simulink library "carnot"  (R2013b)
settings: Solver=ode45  StartTime=0.0  StopTime=10.0  RelTol=1e-3
undefined symbols (not defined in the file or in its folder): A, acol, Ahabit, Awin, Azimuth_Angle, AziWin, B, C, c1, c4, capc, caph, CarnotCallbacks_Density, CarnotCallbacks_Enthalpy, CarnotCallbacks_Enthalpy2Temperature, CarnotCallbacks_Entropy, CarnotCallbacks_Evaporation_Enthalpy, CarnotCallbacks_GlobalMessageLevel, CarnotCallbacks_Grashof, CarnotCallbacks_Heat_Capacity, CarnotCallbacks_Kinematic_Viscosity, CarnotCallbacks_Prandtl, CarnotCallbacks_Saturation_Property, CarnotCallbacks_Saturation_Temperature, CarnotCallbacks_Saturation_Value_Water, CarnotCallbacks_Specific_Volume, CarnotCallbacks_Thermal_Conductivity, CarnotCallbacks_Vapour_Content, CarnotCallbacks_Vapour_Pressure, con, cond, d, Dd, density, dfin, dia, DiameterLastPiece, DPConstant, dpipe, DPLinear, DPQuadratic, emission_out, fluid, FluidMix, FluidType, FPC, frame, g, GeodeticHeight, Gwin, heat_capacity, hgt, HP, Hroom, ID, inlet, K, l, lin, lpipe ... (+29)
undefined symbols (not defined in the file): c2, c3, c5, c6, cwall, dactive, height, mc, mID, rho, tau, UAneighbour, UAwall, uloss
libraries: carnot x333, simulink x25, simulink_extras x7
(part 9 of 16)

== system carnot/Basic/Material_Properties/Entropy ==
  T : Inport
  p : Inport  Port=2
  Fluid_Type : Inport  Port=3
  Fluid_Mix : Inport  Port=4
  SFunction : S-Function  FunctionName=entroflu  Parameters=DEBUGLEVEL,MAXTOTALMESSAGES,MAXCONSECUTIVEMESSAGES,WRITETOFILE,FILENAME  EnableBusSupport=off
  entropy : Outport
  wires:
  SFunction/1 -> entropy/1
  T/1 -> SFunction/3
  p/1 -> SFunction/4
  Fluid_Type/1 -> SFunction/1
  Fluid_Mix/1 -> SFunction/2

== system carnot/Basic/Material_Properties/Evaporation_Enthalpy ==
  T : Inport
  p : Inport  Port=2
  Fluid_Type : Inport  Port=3
  Fluid_Mix : Inport  Port=4
  SFunction : S-Function  FunctionName=evapoent  Parameters=DEBUGLEVEL,MAXTOTALMESSAGES,MAXCONSECUTIVEMESSAGES,WRITETOFILE,FILENAME  EnableBusSupport=off
  evap_enthalpy : Outport
  wires:
  SFunction/1 -> evap_enthalpy/1
  T/1 -> SFunction/3
  p/1 -> SFunction/4
  Fluid_Type/1 -> SFunction/1
  Fluid_Mix/1 -> SFunction/2

== system carnot/Basic/Material_Properties/Heat_Capacity ==
  T : Inport
  p : Inport  Port=2
  Fluid_Type : Inport  Port=3
  Fluid_Mix : Inport  Port=4
  SFunction : S-Function  FunctionName=capfluid  Parameters=DEBUGLEVEL-1,MAXTOTALWARNINGS,MAXCONSECUTIVEWARNINGS,WRITETOFILE,FILENAME  EnableBusSupport=off
  cp : Outport
  wires:
  SFunction/1 -> cp/1
  T/1 -> SFunction/3
  p/1 -> SFunction/4
  Fluid_Type/1 -> SFunction/1
  Fluid_Mix/1 -> SFunction/2

== system carnot/Basic/Material_Properties/Input_Air ==
  Fluid_mix : Constant  Value=x
  Fluid_type : Constant  Value=2
  Temp : Constant  Value=T
  pres : Constant  Value=p
  Temperature : Outport
  Pressure : Outport  Port=2
  Fluid_type: air : Outport  Port=3
  absolute_humidity : Outport  Port=4
  wires:
  Fluid_mix/1 -> absolute_humidity/1
  Fluid_type/1 -> Fluid_type: air/1
  Temp/1 -> Temperature/1
  pres/1 -> Pressure/1

== system carnot/Basic/Material_Properties/Input_Cotton_Oil ==
  Fluid_mix : Constant  Value=0
  Fluid_type : Constant  Value=3
  Temp : Constant  Value=T
  pres : Constant  Value=p
  Temperature : Outport
  Pressure : Outport  Port=2
  Fluid_cotton_oil : Outport  Port=3
  mix : Outport  Port=4
  wires:
  pres/1 -> Pressure/1
  Temp/1 -> Temperature/1
  Fluid_type/1 -> Fluid_cotton_oil/1
  Fluid_mix/1 -> mix/1

== system carnot/Basic/Material_Properties/Input_Fluid ==
  Fluid_mix_ : Constant  Value=x
  Fluid_type_ : Constant  Value=fluid
  Temp : Constant  Value=T
  pres : Constant  Value=p
  Temperature : Outport
  Pressure : Outport  Port=2
  Fluid_type : Outport  Port=3
  Fluid_mix : Outport  Port=4
  wires:
  pres/1 -> Pressure/1
  Temp/1 -> Temperature/1
  Fluid_type_/1 -> Fluid_type/1
  Fluid_mix_/1 -> Fluid_mix/1

== system carnot/Basic/Material_Properties/Input_Silicon_Oil ==
  Fluid_mix : Constant  Value=0
  Fluid_type : Constant  Value=4
  Temp : Constant  Value=T
  pres : Constant  Value=p
  Temperature : Outport
  Pressure : Outport  Port=2
  Fluid_silicon_oil : Outport  Port=3
  mix : Outport  Port=4
  wires:
  Fluid_mix/1 -> mix/1
  Fluid_type/1 -> Fluid_silicon_oil/1
  Temp/1 -> Temperature/1
  pres/1 -> Pressure/1

== system carnot/Basic/Material_Properties/Input_Tyfocor_LS ==
  Fluid_mix : Constant  Value=0
  Fluid_type : Constant  Value=6
  Temp : Constant  Value=T
  pres : Constant  Value=p
  Temperature : Outport
  Pressure : Outport  Port=2
  Fluid_TyfocorLS : Outport  Port=3
  mix : Outport  Port=4
  wires:
  pres/1 -> Pressure/1
  Temp/1 -> Temperature/1
  Fluid_type/1 -> Fluid_TyfocorLS/1
  Fluid_mix/1 -> mix/1

== system carnot/Basic/Material_Properties/Input_Water ==
  Fluid_mix : Constant  Value=xd
  Fluid_type : Constant
  Temp : Constant  Value=T
  pres : Constant  Value=p
  Temperature : Outport
  Pressure : Outport  Port=2
  Fluid_type: water : Outport  Port=3
  vapour_content : Outport  Port=4
  wires:
  pres/1 -> Pressure/1
  Temp/1 -> Temperature/1
  Fluid_type/1 -> Fluid_type: water/1
  Fluid_mix/1 -> vapour_content/1

== system carnot/Basic/Material_Properties/Input_Water_Glycol ==
  Fluid_mix : Constant  Value=g
  Fluid_type : Constant  Value=5
  Temp : Constant  Value=T
  pres : Constant  Value=p
  Temperature : Outport
  Pressure : Outport  Port=2
  Fluid_type: water/glycol : Outport  Port=3
  "volume content of glycol " : Outport  Port=4
  wires:
  pres/1 -> Pressure/1
  Temp/1 -> Temperature/1
  Fluid_type/1 -> Fluid_type: water/glycol/1
  Fluid_mix/1 -> "volume content of glycol "/1

== system carnot/Basic/Material_Properties/Kinematic_Viscosity ==
  T : Inport
  p : Inport  Port=2
  Fluid_Type : Inport  Port=3
  Fluid_Mix : Inport  Port=4
  SFunction : S-Function  FunctionName=viscous  Parameters=DEBUGLEVEL,MAXTOTALMESSAGES,MAXCONSECUTIVEMESSAGES,WRITETOFILE,FILENAME  EnableBusSupport=off
  visc : Outport
  wires:
  SFunction/1 -> visc/1
  T/1 -> SFunction/3
  p/1 -> SFunction/4
  Fluid_Type/1 -> SFunction/1
  Fluid_Mix/1 -> SFunction/2

== system carnot/Basic/Material_Properties/PhaseCheck ==
  THBin : Inport
  S-Function : S-Function  FunctionName=phasechk  EnableBusSupport=off
  THB2THV : carnot/Toolbox/THB2THV
  wires:
  THBin/1 -> THB2THV/1
  THB2THV/1 -> S-Function/1

== system carnot/Basic/Material_Properties/RelHum2x ==
  note: RG      f · ps
      |  x  = ----  --------------
      |         RD     p - f · ps
      |
      | RG = 287.1 Nm/kgK (Gas Constant Air)
      | RD = 461.5 Nm/kgK (Gas Constant Water Vapour)
      | x absolute Humudity
      | f relative Humidity
      | pD partial pressure of water vapour
  T : Inport
  p : Inport  Port=2
  rel_hum : Inport  Port=3
  Product : Product  Inputs=*/  SaturateOnIntegerOverflow=on  InputSameDT=on  OutDataTypeStr=Inherit: Same as first input
  Product1 : Product  Inputs=*/  SaturateOnIntegerOverflow=on  InputSameDT=on  OutDataTypeStr=Inherit: Same as first input
  Saturation : Saturate  UpperLimit=inf  LowerLimit=0
  Sum : Sum  Inputs=-+  SaturateOnIntegerOverflow=on  InputSameDT=on  OutDataTypeStr=Inherit: Same as first input
  Vapour_Pressure : carnot/Basic/Material_Properties/Vapour_Pressure  VariantControl=CarlibClassic  INPUTARGUMENTS=state variables (classic)  DEBUGLEVEL=WARNINGLEVEL  MAXTOTALMESSAGES=inf  MAXCONSECUTIVEMESSAGES=inf  WRITETOFILE=0  FILENAME='errors.txt'
  mix : Constant  Value=0
  molar mass fraction : Gain  Gain=287.1/461.5  SaturateOnIntegerOverflow=on  OutDataTypeStr=Inherit: Same as input  ParamDataTypeStr=Inherit: Same as input
  p12 : Constant
  percent2absolute : Gain  Gain=0.01  SaturateOnIntegerOverflow=on  OutDataTypeStr=Inherit: Same as input  ParamDataTypeStr=Inherit: Same as input
  water : Constant
  x : Outport
  wires:
  p/1 -> Product/1
  Product/1 -> Sum/2
  Sum/1 -> Product1/2
  Product1/1 -> molar mass fraction/1
  T/1 -> Vapour_Pressure/1
  water/1 -> Vapour_Pressure/3
  p12/1 -> Vapour_Pressure/2
  mix/1 -> Vapour_Pressure/4
  Vapour_Pressure/1 -> Sum/1, Product1/1
  rel_hum/1 -> percent2absolute/1
  percent2absolute/1 -> Product/2
  molar mass fraction/1 -> Saturation/1
  Saturation/1 -> x/1

== system carnot/Basic/Material_Properties/Saturation_Property ==
  T : Inport
  p : Inport  Port=2
  Fluid_Type : Inport  Port=3
  Fluid_Mix : Inport  Port=4
  SFunction : S-Function  FunctionName=satprop  Parameters=PROPERTY, FLUIDPHASE, DEBUGLEVEL, MAXTOTALMESSAGES, MAXCONSECUTIVEMESSAGES, WRITETOFILE, FILENAME  EnableBusSupport=off
  enthalpy : Outport
  wires:
  SFunction/1 -> enthalpy/1
  T/1 -> SFunction/3
  p/1 -> SFunction/4
  Fluid_Type/1 -> SFunction/1
  Fluid_Mix/1 -> SFunction/2

== system carnot/Basic/Material_Properties/Saturation_Temperature ==
  T : Inport
  p : Inport  Port=2
  Fluid_Type : Inport  Port=3
  Fluid_Mix : Inport  Port=4
  SFunction : S-Function  FunctionName=satutemp  Parameters=DEBUGLEVEL,MAXTOTALMESSAGES,MAXCONSECUTIVEMESSAGES,WRITETOFILE,FILENAME  EnableBusSupport=off
  Tsat : Outport
  wires:
  SFunction/1 -> Tsat/1
  T/1 -> SFunction/3
  p/1 -> SFunction/4
  Fluid_Type/1 -> SFunction/1
  Fluid_Mix/1 -> SFunction/2

== system carnot/Basic/Material_Properties/Saturation_Value_Water ==
  T : Inport
  p : Inport  Port=2
  Fluid_Type : Inport  Port=3
  Fluid_Mix : Inport  Port=4
  property_id : Inport  Port=5
  SFunction : S-Function  FunctionName=satprop_vec  Parameters=DEBUGLEVEL,MAXTOTALMESSAGES,MAXCONSECUTIVEMESSAGES,WRITETOFILE,FILENAME  EnableBusSupport=off
  saturation_vapour : Outport
  saturation_liquid : Outport  Port=2
  wires:
  SFunction/1 -> saturation_vapour/1
  SFunction/2 -> saturation_liquid/1
  T/1 -> SFunction/3
  p/1 -> SFunction/4
  Fluid_Type/1 -> SFunction/1
  Fluid_Mix/1 -> SFunction/2
  property_id/1 -> SFunction/5

== system carnot/Basic/Material_Properties/Specific_Volume ==
  T : Inport
  p : Inport  Port=2
  Fluid_Type : Inport  Port=3
  Fluid_Mix : Inport  Port=4
  SFunction : S-Function  FunctionName=specivol  Parameters=DEBUGLEVEL-1,MAXTOTALWARNINGS,MAXCONSECUTIVEWARNINGS,WRITETOFILE,FILENAME  EnableBusSupport=off
  spec_vol : Outport
  wires:
  SFunction/1 -> spec_vol/1
  T/1 -> SFunction/3
  p/1 -> SFunction/4
  Fluid_Type/1 -> SFunction/1
  Fluid_Mix/1 -> SFunction/2

== system carnot/Basic/Material_Properties/THB_Wet_BulbTemperature ==
  THB_air : Inport
  Bus Selector : BusSelector  OutputSignals=Temperature,Pressure,FluidType,FluidMix
  Compare To Constant : simulink/Logic and Bit Operations/Compare To Constant  relop===  const=2  OutDataTypeStr=uint8  ZeroCross=off
  Constant : Constant
  Gain : Gain  Gain=100
  MinMax : MinMax  Inputs=2
  Product : Product  Inputs=*/  RndMeth=Zero
  Product1 : Product  RndMeth=Zero
  Product2 : Product  RndMeth=Zero
  Saturation : Saturate  UpperLimit=100  LowerLimit=0
  Vapour_Pressure1 : carnot/Basic/Material_Properties/Vapour_Pressure  VariantControl=CarlibClassic  INPUTARGUMENTS=state variables (classic)  DEBUGLEVEL=WARNINGLEVEL  MAXTOTALMESSAGES=inf  MAXCONSECUTIVEMESSAGES=inf  WRITETOFILE=0  FILENAME='errors.txt'
  Vapour_Pressure2 : carnot/Basic/Material_Properties/Vapour_Pressure  VariantControl=CarlibClassic  INPUTARGUMENTS=state variables (classic)  DEBUGLEVEL=WARNINGLEVEL  MAXTOTALMESSAGES=inf  MAXCONSECUTIVEMESSAGES=inf  WRITETOFILE=0  FILENAME='errors.txt'
  WBT Fcn of relHum+DBT : Lookup2D  RowIndex=[0,5,10,15,20,25,30,35,40,45,50,55,60,65,70,75,80,85,90,95,100]  ColumnIndex=[-6,-4,-2,0,2,4,6,8,10,12,14,16,18,20,22,24,26,28,30,32,34,36,38,40]  Table=reshape([-10.3,-10.1,-9.9,-9.3,-9.3,-8.9,-8.8,-8.8,-8.3,-8.2,-8.2,-7.7,-7.7,-7.7,-7.1,-7.1,-7.1,-6.6,-6.6,-6.0,-6,-8.3,-8.1,-7.9,-7.9,-7.8,-7.3,-7.3,-6.8,-6.8,-6.7,-6.2,-6.2,-5.7,-5.7,-5.6,-5.1,-5.1,-4.6,-4.6,-4.6,-4,-7.2,-6.9,-6.7,-6.4,-6.1,-5.9,-5.6,-5.3,-5.0,-4.8,-4.8,-4.2,-4.2,-3.7,-3.7,-3.1,-3.1,-2.6,-2.6,-2.6,-2,-5.6,-5.3,-5.0,-5.0,-4.4,-4.4,-3.9,-3.9,-3.3,-3.3,-2.8,-2.8,-2.2,-2.2,-1.7,-1.7,-1.1,-1.1,-0.6,-0.6,0,-4.5,-4.2,-3.9,-3.6,-3.0,-2.8,-2.4,-1.9,-1.9,-1.3,-1.3,-0.8,-0.6,-0.2,0.1,0.4,0.7,1.1,1.4,1.7,2,-3.4,-3.0,-2.7,-2.1,-1.6,-1.1,-1.0,-0.4,0.0,0.1,0.5,0.8,1.2,1.6,1.9,2.3,2.6,3.0,3.3,3.7,4,-1.9,-1.5,-1.1,-0.7,-0.3,0.1,0.5,0.9,1.3,1.8,2.2,2.6,3.0,3.4,3.8,4.1,4.5,4.9,5.3,5.6,6,-0.8,-0.4,0.1,0.6,1.1,1.5,2.0,2.5,2.9,3.4,3.8,4.3,4.7,5.1,5.6,6.0,6.4,6.8,7.2,7.6,8,0.3,0.8,1.4,1.9,2.5,3.0,3.5,4.0,4.5,5.0,5.5,6.0,6.5,6.9,7.4,7.8,8.3,8.7,9.2,9.6,10,1.4,2.1,2.7,3.3,3.9,4.4,5.0,5.6,6.1,6.6,7.2,7.7,8.2,8.7,9.2,9.7,10.2,10.6,11.1,11.6,12,2.6,3.2,3.9,4.6,5.2,5.8,6.5,7.1,7.7,8.2,8.8,9.4,9.9,10.5,11.0,11.5,12.0,12.5,13.0,13.5,14,3.7,4.4,5.1,5.9,6.6,7.3,7.9,8.6,9.2,9.9,10.5,11.1,11.7,12.2,12.8,13.4,13.9,14.5,15.0,15.5,16,4.7,5.5,6.3,7.1,7.9,8.6,9.4,10.1,10.8,11.5,12.1,12.8,13.4,14.0,14.6,15.2,15.8,16.4,16.9,17.5,18,5.7,6.6,7.5,8.4,9.2,10.0,10.8,11.6,12.3,13.1,13.8,14.5,15.1,15.8,16.4,17.1,17.7,18.3,18.9,19.4,20,6.7,7.7,8.7,9.6,10.5,11.4,12.2,13.1,13.9,14.6,15.4,16.1,16.9,17.6,18.2,18.9,19.6,20.2,20.8,21.4,22,7.7,8.8,9.8,10.8,11.8,12.8,13.7,14.6,15.4,16.2,17.0,17.8,18.6,19.3,20.1,20.8,21.4,22.1,22.7,23.4,24,8.6,9.8,11.0,12.1,13.1,14.1,15.1,16.0,17.0,17.8,18.7,19.5,20.3,21.1,21.9,22.6,23.3,24.0,24.7,25.4,26,9.6,10.8,12.1,13.3,14.4,15.5,16.5,17.5,18.5,19.4,20.3,21.2,22.1,22.9,23.7,24.5,25.2,25.9,26.6,27.3,28,10.4,11.8,13.2,14.4,15.7,16.8,17.9,19.0,20.0,21.0,22.0,22.9,23.8,24.7,25.5,26.3,27.1,27.8,28.6,29.3,30,11.3,12.8,14.3,15.6,16.9,18.2,19.4,20.5,21.6,22.6,23.6,24.6,25.5,26.4,27.3,28.2,29.0,29.8,30.5,31.3,32,12.1,13.8,15.3,16.8,18.2,19.5,20.8,22.0,23.1,24.2,25.3,26.3,27.3,28.2,29.1,30.0,30.9,31.7,32.5,33.3,34,12.9,14.7,16.4,18.0,19.5,20.9,22.2,23.5,24.7,25.9,27.0,28.0,29.0,30.0,31.0,31.9,32.8,33.6,34.4,35.2,36,13.7,15.7,17.5,19.1,20.7,22.2,23.6,25.0,26.3,27.5,28.6,29.7,30.8,31.8,32.8,33.7,34.7,35.5,36.4,37.2,38,14.5,16.6,18.5,20.3,22.0,23.6,25.1,26.5,27.8,29.1,30.3,31.5,32.6,33.6,34.6,35.6,36.6,37.5,38.3,39.2,40],21,24)  RndMeth=Nearest  LUTDesignDataSource=Matlab Workspace  LUTDesignUseExistingBP=off  LUTDesignAbsError=NaN
  WBT : Outport
  rel_hum : Outport  Port=2
  wires:
  Compare To Constant/1 -> Product1/2, Product2/2
  Product2/1 -> WBT/1
  Product1/1 -> rel_hum/1
  Saturation/1 -> Product1/1, WBT Fcn of relHum+DBT/1
  Gain/1 -> Saturation/1
  WBT Fcn of relHum+DBT/1 -> Product2/1
  Product/1 -> Gain/1
  MinMax/1 -> Product/1
  Vapour_Pressure2/1 -> Product/2, MinMax/2
  Vapour_Pressure1/1 -> MinMax/1
  Constant/1 -> Vapour_Pressure2/3, Vapour_Pressure2/4
  Bus Selector/1 -> Vapour_Pressure1/1, Vapour_Pressure2/1, WBT Fcn of relHum+DBT/2  "<Temperature>"
  Bus Selector/4 -> Vapour_Pressure1/4  "<FluidMix>"
  Bus Selector/3 -> Compare To Constant/1, Vapour_Pressure1/3  "<FluidType>"
  Bus Selector/2 -> Vapour_Pressure1/2, Vapour_Pressure2/2  "<Pressure>"
  THB_air/1 -> Bus Selector/1

== system carnot/Basic/Material_Properties/Thermal_Conductivity ==
  T : Inport
  p : Inport  Port=2
  Fluid_Type : Inport  Port=3
  Fluid_Mix : Inport  Port=4
  SFunction : S-Function  FunctionName=conduct  Parameters=DEBUGLEVEL,MAXTOTALMESSAGES,MAXCONSECUTIVEMESSAGES,WRITETOFILE,FILENAME  EnableBusSupport=off
  cond : Outport
  wires:
  SFunction/1 -> cond/1
  T/1 -> SFunction/3
  p/1 -> SFunction/4
  Fluid_Type/1 -> SFunction/1
  Fluid_Mix/1 -> SFunction/2

== system carnot/Basic/Material_Properties/Vapour_Content ==
  T : Inport
  p : Inport  Port=2
  Fluid_Type : Inport  Port=3
  Fluid_Mix : Inport  Port=4
  value : Inport  Port=5
  SFunction : S-Function  FunctionName=vapocont  Parameters=PROPERTYTYPE, DEBUGLEVEL, MAXTOTALMESSAGES, MAXCONSECUTIVEMESSAGES,WRITETOFILE, FILENAME  EnableBusSupport=off
  vapcont : Outport
  wires:
  SFunction/1 -> vapcont/1
  T/1 -> SFunction/3
  p/1 -> SFunction/4
  Fluid_Type/1 -> SFunction/1
  Fluid_Mix/1 -> SFunction/2
  value/1 -> SFunction/5

== system carnot/Basic/Material_Properties/Vapour_Pressure ==
  T : Inport
  p : Inport  Port=2
  Fluid_Type : Inport  Port=3
  Fluid_Mix : Inport  Port=4
  SFunction : S-Function  FunctionName=vappress  Parameters=DEBUGLEVEL,MAXTOTALMESSAGES,MAXCONSECUTIVEMESSAGES,WRITETOFILE,FILENAME  EnableBusSupport=off
  vappress : Outport
  wires:
  SFunction/1 -> vappress/1
  T/1 -> SFunction/3
  p/1 -> SFunction/4
  Fluid_Type/1 -> SFunction/1
  Fluid_Mix/1 -> SFunction/2

== system carnot/Basic/Material_Properties/x2RelHum ==
  note: x · p
      | f =  -----------------
      |         ps ( RG/RD + x)
      |
      | RG = 287.1 Nm/kgK (Gas Constant Air)
      | RD = 461.5 Nm/kgK (Gas Constant Water Vapour)
      | x absolute Humudity
      | f relative Humidity
      | pD partial pressure of water vapour
  T : Inport
  p : Inport  Port=2
  x : Inport  Port=3
  Product1 : Product  Inputs=//**  SaturateOnIntegerOverflow=on  InputSameDT=on  OutDataTypeStr=Inherit: Same as first input
  Saturation : Saturate  UpperLimit=100  LowerLimit=0
  Sum : Sum  Inputs=|++  SaturateOnIntegerOverflow=on  InputSameDT=on  OutDataTypeStr=Inherit: Same as first input
  Vapour_Pressure : carnot/Basic/Material_Properties/Vapour_Pressure  VariantControl=CarlibClassic  INPUTARGUMENTS=state variables (classic)  DEBUGLEVEL=WARNINGLEVEL  MAXTOTALMESSAGES=inf  MAXCONSECUTIVEMESSAGES=inf  WRITETOFILE=0  FILENAME='errors.txt'
  mix : Constant  Value=0
  "molar mass fraction " : Constant  Value=287.1/461.5
  p12 : Constant
  to percent : Gain  Gain=100  SaturateOnIntegerOverflow=on  OutDataTypeStr=Inherit: Same as input  ParamDataTypeStr=Inherit: Same as input
  water : Constant
  rel_hum : Outport
  wires:
  mix/1 -> Vapour_Pressure/4
  p12/1 -> Vapour_Pressure/2
  water/1 -> Vapour_Pressure/3
  T/1 -> Vapour_Pressure/1
  Product1/1 -> to percent/1
  x/1 -> Sum/2, Product1/4
  p/1 -> Product1/3
  Sum/1 -> Product1/2
  Vapour_Pressure/1 -> Product1/1
  to percent/1 -> Saturation/1
  Saturation/1 -> rel_hum/1
  "molar mass fraction "/1 -> Sum/1

== system carnot/Basic/Pressure_Drop/Pressure_Drop_Collector ==
  Tnodes : Inport
  THBin : Inport  Port=2
  position : Inport  Port=3
  Bus Selector3 : BusSelector  OutputSignals=inclination
  Degrees to Radians : simulink_extras/Transformations/Degrees to Radians
  Gain : Gain  Gain=len
  Pressure_Drop_Fix : carnot/Basic/Pressure_Drop/Pressure_Drop_Fix  con=0  lin=lin  qua=qua
  Pressure_Drop_staticHeight : carnot/Basic/Pressure_Drop/Pressure_Drop_staticHeight
  Trigonometric Function : Trigonometry
  THB : Outport
  wires:
  Degrees to Radians/1 -> Trigonometric Function/1
  Gain/1 -> Pressure_Drop_staticHeight/3
  Pressure_Drop_staticHeight/1 -> THB/1
  Tnodes/1 -> Pressure_Drop_staticHeight/1
  Pressure_Drop_Fix/1 -> Pressure_Drop_staticHeight/2
  THBin/1 -> Pressure_Drop_Fix/1
  Trigonometric Function/1 -> Gain/1
  position/1 -> Bus Selector3/1
  Bus Selector3/1 -> Degrees to Radians/1  "<inclination>"

== system carnot/Basic/Pressure_Drop/Pressure_Drop_Fix ==
  THB : Inport
  Abs : Abs
  Bus Assignment1 : BusAssignment  AssignedSignals=Pressure,DPConstant,DPLinear,DPQuadratic
  Bus Selector3 : BusSelector  OutputSignals=MassFlow,Pressure
  Bus Selector4 : BusSelector  OutputSignals=DPConstant,DPLinear,DPQuadratic  OutputAsBus=on
  Bus Selector5 : BusSelector  OutputSignals=ID
  Compare To Constant1 : simulink/Logic and Bit Operations/Compare To Constant  relop=>  const=10000  OutDataTypeStr=boolean
  Compare To Constant2 : simulink/Logic and Bit Operations/Compare To Constant  relop=>  const=20000  OutDataTypeStr=boolean
  Demux2 : Demux  Outputs=3
  Pressuredrop : carnot/Basic/Pressure_Drop/Pressuredrop
  Terminator1 : Terminator
  c_calc : Subsystem
  lq_calc : Subsystem
  THB_ : Outport
  wires:
  Pressuredrop/3 -> Terminator1/1
  Pressuredrop/2 -> Demux2/1
  c_calc/1(con) -> Pressuredrop/4
  Compare To Constant2/1 -> c_calc/Enable
  Bus Selector5/1 -> Abs/1  "<ID>"
  Bus Selector3/2 -> Pressuredrop/2  "<Pressure>"
  Bus Selector3/1 -> Pressuredrop/1  "<MassFlow>"
  Bus Selector4/1 -> Pressuredrop/3
  Abs/1 -> Compare To Constant1/1, Compare To Constant2/1
  THB/1 -> Bus Selector5/1, Bus Selector3/1, Bus Selector4/1, Bus Assignment1/1
  Pressuredrop/1 -> Bus Assignment1/2
  Bus Assignment1/1 -> THB_/1
  Demux2/1 -> Bus Assignment1/3
  Demux2/2 -> Bus Assignment1/4
  Demux2/3 -> Bus Assignment1/5
  lq_calc/1(Out1) -> Pressuredrop/5
  lq_calc/2(Out2) -> Pressuredrop/6
  Compare To Constant1/1 -> lq_calc/Enable

== matlab function carnot/Source/Chiller/Cooling_Tower/Feuchtkugel- temperatureinfluss // wet-bulb temperature effect/Abgleich /Embedded MATLAB Function ==
  data: t_fk input; y output; t_ia_fk15 input; t_ie input
%Festlegung der Eingänge
function y = fcn(t_fk, t_ia_fk15, t_ie)

%Änderung des Faktors
if t_ie < 41
    
    y = ((t_fk-15)*0.27)+t_ia_fk15;
    
else
    
    y = ((t_fk-15)*0.25)+t_ia_fk15;
    
end

== matlab function carnot/Source/Chiller/Cooling_Tower/Leistungseinflüsse // influence on coolingpower/t_ia_ist /isinf ==
  data: u input; y output

function y = fcn(u)

%Verhindert die Fehlerausgabe bei Teilen mit dem Wert 0 
%Dieser Zustand tritt ein wenn der Volumenstrom 0 l/s gesetzt wird.

v = isinf (u);

if v == 0
    
    y = u;

else 
    
    y = 0;
    
end

== matlab function carnot/Source/Chiller/Cooling_Tower/Verbrauch // consumption/Verdunstung/Verdunstungsmenge ==
  data: h_le input; mdot input; x_fl output; qdot input; t_ie input; x_le input; t_tau input; p input
function x_fl = fcn(h_le, mdot, qdot, t_ie, x_le, t_tau, p)

cp_lt = 1.006;
cp_d = 1.861;
cp_w = 4.19;
dhv0 = 2500;
tmax = t_ie;
tmin = t_tau;
t_zw = 15;
phi_luftaus = 100;
m = 1;


% Vorbedingung qdot muss positiv sein um eine Verdunstung zu gewährleisten ansonsten ist es ein Kondensation
if qdot < 0
    
    x_luftaus = 0;
    
else
    % Luftaustrittstemperaturberechnung, Halbierungsverfahren
        t_luftaus = (tmax+tmin)/2;
    
    % Absolute Feuchte-Berechnung Lufteintritt
        ps_luftaus = 611*exp((-1.91275)*10^(-4)+7.258*10^(-2)*t_luftaus-2.939*10^(-4)*t_luftaus^2+9.841*10^(-7)*t_luftaus^3-1.92*10^(-9)*t_luftaus^4);
        x_luftaus = (0.622*(phi_luftaus/100)*ps_luftaus)/(p-(phi_luftaus/100)*ps_luftaus);

    % Enthalpie Luftaustritt mit dem schon berechneten Qpkt
        h_la = qdot/mdot + (x_luftaus-x_le)*cp_w*t_zw + h_le;
    
    % Austrittstemperatur 
        tlab = (h_la - x_luftaus*dhv0)/(cp_lt + x_luftaus*cp_d);

    % Beginn der Schleife 
    % (t_luftaus - tlab) < 0,001 und > -0,001 ist die Austrittstemperatur gefunden
    %  t_luftaus < tlab  tmin = t_luftaus
    %  t_luftaus > tlab  tmax = t_luftaus
        while (t_luftaus - tlab)>0.001 || (t_luftaus - tlab) < -0.001 && m < 30
    
            if t_luftaus < tlab
        
                tmin = t_luftaus;
    
            else
        
                tmax = t_luftaus;
    
            end
    
            % Luftaustrittstemperaturberechnung, Halbierungsverfahren
                t_luftaus = (tmax+tmin)/2;
    
            % Absolute Feuchte-Berechnung Lufteintritt
                ps_luftaus = 611*exp((-1.91275)*10^(-4)+7.258*10^(-2)*t_luftaus-2.939*10^(-4)*t_luftaus^2+9.841*10^(-7)*t_luftaus^3-1.92*10^(-9)*t_luftaus^4);
                x_luftaus = (0.622*(phi_luftaus/100)*ps_luftaus)/(p-(phi_luftaus/100)*ps_luftaus);
        
            % Enthalpie Luftaustritt mit dem schon berechneten Qpkt
                h_la = qdot/mdot + (x_luftaus-x_le)*cp_w*t_zw + h_le;
        
            % Austrittstemperatur 
                tlab = (h_la - x_luftaus*dhv0)/(cp_lt + x_luftaus*cp_d);
        
            % Schleifenzähler
                m = m + 1;
    
        end

end

x_fl = x_luftaus-x_le;

== system carnot/Basic/Pressure_Drop/Pressure_Drop_PipeTheory ==
  Tnodes : Inport
  THBin : Inport  Port=2
  Abs : Abs
  Bus Assignment : BusAssignment  AssignedSignals=Pressure,DPConstant,DPLinear,DPQuadratic
  Bus Selector : BusSelector  OutputSignals=MassFlow,Pressure
  Bus Selector1 : BusSelector  OutputSignals=DPConstant,DPLinear,DPQuadratic  OutputAsBus=on
  Bus Selector2 : BusSelector  OutputSignals=ID
  Compare To Constant1 : simulink/Logic and Bit Operations/Compare To Constant  relop=>  const=10000  OutDataTypeStr=boolean
  DP_Geometry : Subsystem
  Demux : Demux  Outputs=3
  Pressuredrop : carnot/Basic/Pressure_Drop/Pressuredrop
  Terminator : Terminator
  Terminator1 : Terminator
  const1 : Constant  Value=0
  THB : Outport
  wires:
  DP_Geometry/3(dp) -> Terminator1/1
  DP_Geometry/2(qua) -> Pressuredrop/6
  DP_Geometry/1(lin) -> Pressuredrop/5
  Pressuredrop/2 -> Demux/1
  Demux/3 -> Bus Assignment/5
  Demux/2 -> Bus Assignment/4
  Demux/1 -> Bus Assignment/3
  Pressuredrop/1 -> Bus Assignment/2
  Bus Assignment/1 -> THB/1
  THBin/1 -> Bus Selector/1, Bus Selector1/1, Bus Selector2/1, DP_Geometry/2(mdot), Bus Assignment/1
  Abs/1 -> Compare To Constant1/1
  Bus Selector1/1 -> Pressuredrop/3
  Bus Selector/1 -> Pressuredrop/1  "<MassFlow>"
  Bus Selector/2 -> Pressuredrop/2  "<Pressure>"
  Bus Selector2/1 -> Abs/1  "<ID>"
  Tnodes/1 -> DP_Geometry/1(Tnodes)
  Compare To Constant1/1 -> DP_Geometry/Enable
  Pressuredrop/3 -> Terminator/1
  const1/1 -> Pressuredrop/4

== system carnot/Basic/Pressure_Drop/Pressure_Drop_StorageHX ==
  THBin : Inport
  Bus Selector : BusSelector  OutputSignals=Temperature
  Constant : Constant  Value=hgt
  Pressure_Drop_Fix : carnot/Basic/Pressure_Drop/Pressure_Drop_Fix  con=0  lin=dplin  qua=dpqua
  Pressure_Drop_changeD : carnot/Basic/Pressure_Drop/Pressure_Drop_changeD  dia=dia
  Pressure_Drop_staticHeight : carnot/Basic/Pressure_Drop/Pressure_Drop_staticHeight
  THB : Outport
  wires:
  Pressure_Drop_staticHeight/1 -> Pressure_Drop_Fix/1
  Pressure_Drop_changeD/1 -> Pressure_Drop_staticHeight/2
  Constant/1 -> Pressure_Drop_staticHeight/3
  THBin/1 -> Pressure_Drop_changeD/1, Bus Selector/1
  Bus Selector/1 -> Pressure_Drop_staticHeight/1  "<Temperature>"
  Pressure_Drop_Fix/1 -> THB/1

== system carnot/Basic/Pressure_Drop/Pressure_Drop_StoragePipe ==
  Tnodes : Inport
  THBin : Inport  Port=2
  Constant : Constant  Value=hgt
  Pressure_Drop_changeD : carnot/Basic/Pressure_Drop/Pressure_Drop_changeD  dia=dia
  Pressure_Drop_staticHeight : carnot/Basic/Pressure_Drop/Pressure_Drop_staticHeight
  THB : Outport
  wires:
  THBin/1 -> Pressure_Drop_changeD/1
  Constant/1 -> Pressure_Drop_staticHeight/3
  Pressure_Drop_changeD/1 -> Pressure_Drop_staticHeight/2
  Tnodes/1 -> Pressure_Drop_staticHeight/1
  Pressure_Drop_staticHeight/1 -> THB/1

== system carnot/Basic/Pressure_Drop/Pressure_Drop_changeD ==
  THBin : Inport
  2/pi/d^2/density : Subsystem
  Abs : Abs
  Bus Assignment : BusAssignment  AssignedSignals=Pressure,DPConstant,DPLinear,DPQuadratic,DiameterLastPiece
  Bus Selector : BusSelector  OutputSignals=MassFlow,Pressure
  Bus Selector1 : BusSelector  OutputSignals=DPConstant,DPLinear,DPQuadratic  OutputAsBus=on
  Bus Selector2 : BusSelector  OutputSignals=ID
  Compare To Constant1 : simulink/Logic and Bit Operations/Compare To Constant  relop=>  const=10000  OutDataTypeStr=boolean
  Constant : Constant  Value=0
  Demux : Demux  Outputs=3
  Pressuredrop : carnot/Basic/Pressure_Drop/Pressuredrop
  Terminator : Terminator
  diameter : Constant  Value=dia
  THB : Outport
  wires:
  diameter/1 -> Bus Assignment/6
  Pressuredrop/2 -> Demux/1
  Demux/3 -> Bus Assignment/5
  Demux/2 -> Bus Assignment/4
  Demux/1 -> Bus Assignment/3
  Pressuredrop/1 -> Bus Assignment/2
  Bus Assignment/1 -> THB/1
  THBin/1 -> Bus Assignment/1, Bus Selector/1, Bus Selector1/1, Bus Selector2/1, 2/pi/d^2/density/1(THB)
  Abs/1 -> Compare To Constant1/1
  Bus Selector1/1 -> Pressuredrop/3
  Bus Selector/1 -> Pressuredrop/1  "<MassFlow>"
  Bus Selector/2 -> Pressuredrop/2  "<Pressure>"
  Bus Selector2/1 -> Abs/1  "<ID>"
  Constant/1 -> Pressuredrop/5, Pressuredrop/4
  2/pi/d^2/density/1(qua) -> Pressuredrop/6
  Compare To Constant1/1 -> 2/pi/d^2/density/Enable
  Pressuredrop/3 -> Terminator/1

== system carnot/Basic/Pressure_Drop/Pressure_Drop_staticHeight ==
  Tnodes : Inport
  THBin : Inport  Port=2
  height : Inport  Port=3
  Abs : Abs
  Bus Assignment : BusAssignment  AssignedSignals=Pressure,DPConstant,DPLinear,DPQuadratic,GeodeticHeight
  Bus Selector : BusSelector  OutputSignals=MassFlow,Pressure
  Bus Selector1 : BusSelector  OutputSignals=DPConstant,DPLinear,DPQuadratic  OutputAsBus=on
  Bus Selector2 : BusSelector  OutputSignals=ID
  Compare To Constant : simulink/Logic and Bit Operations/Compare To Constant  relop=>  const=20000  OutDataTypeStr=boolean
  Demux : Demux  Outputs=3
  Density_x_Gravity : Subsystem
  Pressuredrop : carnot/Basic/Pressure_Drop/Pressuredrop
  Terminator : Terminator
  const1 : Constant  Value=0
  const2 : Constant  Value=0
  THB : Outport
  wires:
  Density_x_Gravity/2(GeodeticHeight) -> Bus Assignment/6
  height/1 -> Density_x_Gravity/3(height)
  Pressuredrop/2 -> Demux/1
  Demux/3 -> Bus Assignment/5
  Demux/2 -> Bus Assignment/4
  Demux/1 -> Bus Assignment/3
  Pressuredrop/1 -> Bus Assignment/2
  Bus Assignment/1 -> THB/1
  THBin/1 -> Bus Assignment/1, Bus Selector/1, Bus Selector1/1, Density_x_Gravity/2(THB), Bus Selector2/1
  Abs/1 -> Compare To Constant/1
  Bus Selector1/1 -> Pressuredrop/3
  Bus Selector/1 -> Pressuredrop/1  "<MassFlow>"
  Bus Selector/2 -> Pressuredrop/2  "<Pressure>"
  Bus Selector2/1 -> Abs/1  "<ID>"
  Tnodes/1 -> Density_x_Gravity/1(Tnodes)
  Compare To Constant/1 -> Density_x_Gravity/Enable
  Density_x_Gravity/1(pstat) -> Pressuredrop/4
  Pressuredrop/3 -> Terminator/1
  const1/1 -> Pressuredrop/5
  const2/1 -> Pressuredrop/6

== system carnot/Basic/Pressure_Drop/Pressuredrop ==
  mdot : Inport
  p_in : Inport  Port=2
  clq_in : Inport  Port=3
  con : Inport  Port=4
  lin : Inport  Port=5
  qua : Inport  Port=6
  Constant : Constant
  Dot Product : DotProduct  InputSameDT=on  OutDataTypeStr=Inherit: Inherit via internal rule
  Math Function : Math  Operator=square  SaturateOnIntegerOverflow=on
  Mux : Mux  Inputs=3
  Mux1 : Mux  Inputs=3
  Saturation : Saturate  UpperLimit=inf  LowerLimit=0
  sum : Sum  SaturateOnIntegerOverflow=on  InputSameDT=on  OutDataTypeStr=Inherit: Same as first input
  sum1 : Sum  Inputs=+-  SaturateOnIntegerOverflow=on  InputSameDT=on  OutDataTypeStr=Inherit: Same as first input
  p_out : Outport
  clq_out : Outport  Port=2
  dp : Outport  Port=3
  wires:
  sum1/1 -> Saturation/1
  p_in/1 -> sum1/1
  Dot Product/1 -> dp/1, sum1/2
  Mux1/1 -> Dot Product/2, sum/2
  sum/1 -> clq_out/1
  clq_in/1 -> sum/1
  qua/1 -> Mux1/3
  lin/1 -> Mux1/2
  con/1 -> Mux1/1
  Mux/1 -> Dot Product/1
  Math Function/1 -> Mux/3
  mdot/1 -> Math Function/1, Mux/2
  Constant/1 -> Mux/1
  Saturation/1 -> p_out/1

== system carnot/Basic/Thermal_Models/Combustion_Calculation ==
  Qdot_fuel : Inport
  efficiency : Inport  Port=2
  Pelec : Inport  Port=3
  Tm : Inport  Port=4
  fuel : Inport  Port=5
  Enable : EnablePort
  Bus Creator : BusCreator  Inputs=16
  Bus Selector : BusSelector  OutputSignals=Fuel_ID,Pressure,h_Vector,Price,MassFraction_H,MassFraction_C,MassFraction_O,MassFraction_S,MassFraction_N,MassFraction_H2O
  Selector : Selector  IndexOptions=Index vector (dialog)  Indices=[1]  OutputSizes=1
  Signal Conversion : SignalConversion
  exhaust gas : Subsystem
  mdotCO2 : Product  SaturateOnIntegerOverflow=on  InputSameDT=on  OutDataTypeStr=Inherit: Same as first input
  mdotH20 : Product  SaturateOnIntegerOverflow=on  InputSameDT=on  OutDataTypeStr=Inherit: Same as first input
  mdotN2 : Product  SaturateOnIntegerOverflow=on  InputSameDT=on  OutDataTypeStr=Inherit: Same as first input
  mdotNOx : Product  SaturateOnIntegerOverflow=on  InputSameDT=on  OutDataTypeStr=Inherit: Same as first input
  mdotSO2 : Product  SaturateOnIntegerOverflow=on  InputSameDT=on  OutDataTypeStr=Inherit: Same as first input
  mdot_CO : Constant  Value=0
  mdot_CxHy : Constant  Value=0
  mdot_O2 : Constant  Value=0
  n2 : Constant  Value=0
  pricedot : Product  SaturateOnIntegerOverflow=on  InputSameDT=on  OutDataTypeStr=Inherit: Same as first input
  prod : Product  Inputs=*/  SaturateOnIntegerOverflow=on  InputSameDT=on  OutDataTypeStr=Inherit: Same as first input
  eco : Outport  InitialOutput=0
  wires:
  Tm/1 -> Bus Creator/2  "Tmean"
  Qdot_fuel/1 -> Bus Creator/5, prod/1  "Qdot_fuel"
  mdotN2/1 -> Bus Creator/12  "mdotN2"
  exhaust gas/2(H2O) -> mdotH20/2
  exhaust gas/1(CO2) -> mdotCO2/2
  exhaust gas/4(N2) -> mdotN2/2
  n2/1 -> mdotNOx/2
  exhaust gas/3(SO2) -> mdotSO2/2
  Bus Selector/10 -> exhaust gas/7(w)  "<MassFraction_H2O>"
  Bus Selector/9 -> exhaust gas/6(n)  "<MassFraction_N>"
  Bus Selector/8 -> exhaust gas/5(s)  "<MassFraction_S>"
  Bus Selector/7 -> exhaust gas/4(o)  "<MassFraction_O>"
  Bus Selector/6 -> exhaust gas/3(c)  "<MassFraction_C>"
  Bus Selector/5 -> exhaust gas/2(h)  "<MassFraction_H>"
  Bus Selector/2 -> Bus Creator/4  "<Pressure>"
  Bus Selector/1 -> Bus Creator/1, exhaust gas/1(ID)  "<Fuel_ID>"
  prod/1 -> Bus Creator/3, mdotN2/1, mdotNOx/1, mdotSO2/1, mdotCO2/1, mdotH20/1, pricedot/1  "mdot_fuel"
  Bus Selector/4 -> pricedot/2  "<Price>"
  mdot_CxHy/1 -> Bus Creator/15  "mdot_CxHy"
  mdot_CO/1 -> Bus Creator/14  "mdot_CO"
  mdotNOx/1 -> Bus Creator/13  "mdotNOx"
  mdotSO2/1 -> Bus Creator/11  "mdotSO2"
  mdot_O2/1 -> Bus Creator/10  "mdot_O2"
  mdotCO2/1 -> Bus Creator/9  "mdotCO2"
  mdotH20/1 -> Bus Creator/8  "mdotH20"
  pricedot/1 -> Bus Creator/7  "MoneyFlow"
  Pelec/1 -> Bus Creator/6  "Pelec"
  Bus Creator/1 -> Signal Conversion/1
  Bus Selector/3 -> Selector/1  "<h_Vector>"
  fuel/1 -> Bus Selector/1
  efficiency/1 -> Bus Creator/16  "Efficiency"
  Selector/1 -> prod/2
  Signal Conversion/1 -> eco/1

== system carnot/Basic/Thermal_Models/HeatPump_basic ==
  THBin_source : Inport
  THB_in_load : Inport  Port=2
  Tamb : Inport  Port=3
  on/off : Inport  Port=4
  Bus Assignment : BusAssignment  AssignedSignals=Temperature
  Bus Assignment1 : BusAssignment  AssignedSignals=Temperature
  Bus Creator : BusCreator  Inputs=7
  Bus Selector : BusSelector  OutputSignals=Temperature,MassFlow,Pressure,FluidType,FluidMix
  Bus Selector1 : BusSelector  OutputSignals=Temperature,MassFlow,Pressure,FluidType,FluidMix
  P_el calculus : Subsystem
  Product : DotProduct  InputSameDT=on  OutDataTypeStr=Inherit: Inherit via internal rule
  Product1 : DotProduct  InputSameDT=on  OutDataTypeStr=Inherit: Inherit via internal rule
  Product3 : DotProduct  InputSameDT=on  OutDataTypeStr=Inherit: Inherit via internal rule
  Sum1 : Sum  Inputs=+-  SaturateOnIntegerOverflow=on  InputSameDT=on  OutDataTypeStr=Inherit: Same as first input
  Sum2 : Sum  Inputs=+-  SaturateOnIntegerOverflow=on  InputSameDT=on  OutDataTypeStr=Inherit: Same as first input
  model cold side : Subsystem
  model hot side : Subsystem
  THBsource : Outport
  THBload : Outport  Port=2
  data_hp : Outport  Port=3
  wires:
  Product/1 -> Bus Creator/6  "Qdot_hot"
  Product3/1 -> Bus Creator/3  "Qdot_cold"
  model cold side/2(mdot*cp) -> Product3/2
  Sum1/1 -> Product3/1
  Bus Selector1/2 -> model cold side/2(mdot_cold)  "<MassFlow>"
  on/off/1 -> model hot side/8(command), Product1/1, model cold side/8(command)
  model hot side/2(Thot_out) -> Sum2/1, P_el calculus/1(Thot_out), model cold side/6(Thot), Bus Assignment/2
  Product1/1 -> Bus Creator/7  "Pelec"
  P_el calculus/1(P_el) -> Product1/2
  Bus Selector/3 -> model hot side/4(p_hot)  "<Pressure>"
  model cold side/1(Tcold_out) -> Bus Assignment1/2, Sum1/2
  Bus Selector1/1 -> model cold side/1(Tcold), Sum1/1, model hot side/1(Tcold), P_el calculus/2(Tcold_in)  "<Temperature>"
  Sum2/1 -> Product/2
  model hot side/1(mdot*cp) -> Product/1
  Bus Selector/2 -> model hot side/3(mdot_hot)  "<MassFlow>"
  Bus Selector/1 -> model hot side/2(Thot), Sum2/2  "<Temperature>"
  Bus Selector/5 -> model hot side/6(mix_hot)  "<FluidMix>"
  Bus Selector/4 -> model hot side/5(fluid_hot)  "<FluidType>"
  Bus Selector1/3 -> model cold side/3(p_cold)  "<Pressure>"
  Bus Selector1/4 -> model cold side/4(fluid_cold)  "<FluidType>"
  Bus Selector1/5 -> model cold side/5(mix_cold)  "<FluidMix>"
  THB_in_load/1 -> Bus Selector/1, Bus Assignment/1, Bus Creator/4  "THBin_hot"
  Tamb/1 -> model cold side/7(Tamb), model hot side/7(Tamb)
  Bus Assignment/1 -> THBload/1, Bus Creator/5  "THBout_hot"
  THBin_source/1 -> Bus Selector1/1, Bus Assignment1/1, Bus Creator/1  "THBin_cold"
  Bus Assignment1/1 -> THBsource/1, Bus Creator/2  "THBout_cold"
  Bus Creator/1 -> data_hp/1

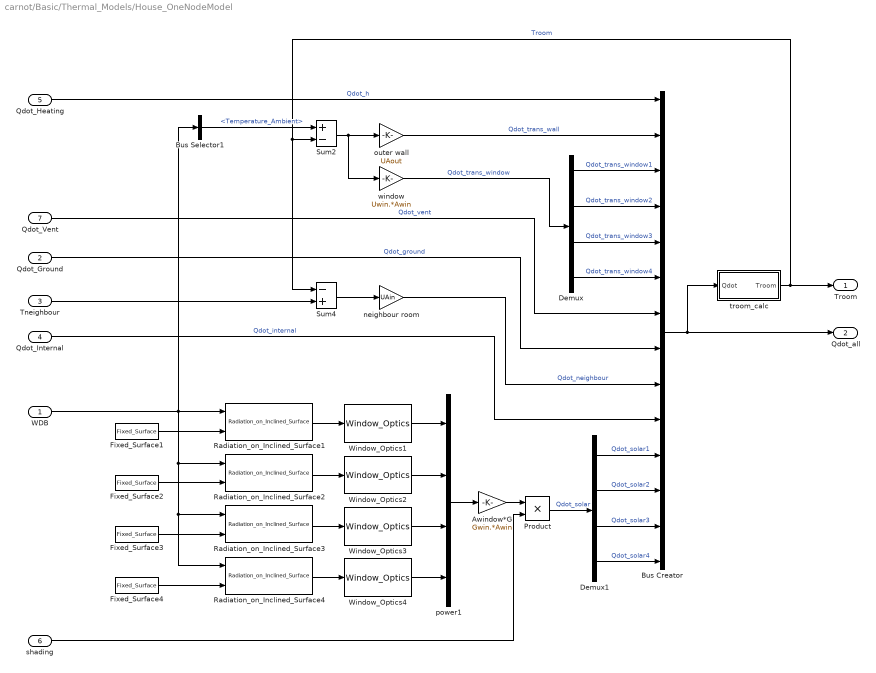
== system carnot/Basic/Thermal_Models/House_OneNodeModel ==
  WDB : Inport
  Qdot_Ground : Inport  Port=2
  Tneighbour : Inport  Port=3
  Qdot_Internal : Inport  Port=4
  Qdot_Heating : Inport  Port=5
  shading : Inport  Port=6
  Qdot_Vent : Inport  Port=7
  Awindow*G : Gain  Gain=Gwin.*Awin  SaturateOnIntegerOverflow=on  OutDataTypeStr=Inherit: Same as input  ParamDataTypeStr=Inherit: Same as input
  Bus Creator : BusCreator  Inputs=14
  Bus Selector1 : BusSelector  OutputSignals=Temperature_Ambient
  Demux : Demux
  Demux1 : Demux
  Fixed_Surface1 : carnot/Weather/Fixed_Surface  colangle=90  colazi=AziWin(1)  colrot=0
  Fixed_Surface2 : carnot/Weather/Fixed_Surface  colangle=90  colazi=AziWin(2)  colrot=0
  Fixed_Surface3 : carnot/Weather/Fixed_Surface  colangle=90  colazi=AziWin(3)  colrot=0
  Fixed_Surface4 : carnot/Weather/Fixed_Surface  colangle=90  colazi=AziWin(4)  colrot=0
  Product : Product  RndMeth=Zero
  Radiation_on_Inclined_Surface{1..4} (4 alike) : carnot/Weather/Radiation_on_Inclined_Surface  sky=Perez 1990  reflect=0.2
  Sum2 : Sum  Inputs=+-  SaturateOnIntegerOverflow=on  InputSameDT=on  OutDataTypeStr=Inherit: Same as first input
  Sum4 : Sum  Inputs=-+  SaturateOnIntegerOverflow=on  InputSameDT=on  OutDataTypeStr=Inherit: Same as first input
  Window_Optics{1..4} (4 alike) : carnot/Load/Houses/wall_floor/Window_Optics
  neighbour room : Gain  Gain=UAin  SaturateOnIntegerOverflow=on  OutDataTypeStr=Inherit: Same as input  ParamDataTypeStr=Inherit: Same as input
  outer wall : Gain  Gain=UAout  SaturateOnIntegerOverflow=on  OutDataTypeStr=Inherit: Same as input  ParamDataTypeStr=Inherit: Same as input
  power1 : Mux
  troom_calc : Subsystem
  window : Gain  Gain=Uwin.*Awin  SaturateOnIntegerOverflow=on  OutDataTypeStr=Inherit: Same as input  ParamDataTypeStr=Inherit: Same as input
  Troom : Outport
  Qdot_all : Outport  Port=2
  wires:
  Tneighbour/1 -> Sum4/2
  Qdot_Vent/1 -> Bus Creator/7  "Qdot_vent"
  shading/1 -> Product/2
  Awindow*G/1 -> Product/1
  Qdot_Heating/1 -> Bus Creator/1  "Qdot_h"
  Window_Optics4/1 -> power1/4
  Window_Optics3/1 -> power1/3
  Window_Optics2/1 -> power1/2
  Window_Optics1/1 -> power1/1
  Product/1 -> Demux1/1  "Qdot_solar"
  Sum2/1 -> outer wall/1, window/1
  outer wall/1 -> Bus Creator/2  "Qdot_trans_wall"
  Bus Selector1/1 -> Sum2/1  "<Temperature_Ambient>"
  WDB/1 -> Radiation_on_Inclined_Surface3/1, Radiation_on_Inclined_Surface4/1, Radiation_on_Inclined_Surface2/1, Radiation_on_Inclined_Surface1/1, Bus Selector1/1
  Bus Creator/1 -> troom_calc/1(Qdot), Qdot_all/1
  Qdot_Ground/1 -> Bus Creator/8  "Qdot_ground"
  Sum4/1 -> neighbour room/1
  Demux/1 -> Bus Creator/3  "Qdot_trans_window1"
  neighbour room/1 -> Bus Creator/9  "Qdot_neighbour"
  Qdot_Internal/1 -> Bus Creator/10  "Qdot_internal"
  Fixed_Surface1/1 -> Radiation_on_Inclined_Surface1/2
  Radiation_on_Inclined_Surface1/1 -> Window_Optics1/1
  power1/1 -> Awindow*G/1
  Fixed_Surface2/1 -> Radiation_on_Inclined_Surface2/2
  Radiation_on_Inclined_Surface2/1 -> Window_Optics2/1
  Fixed_Surface3/1 -> Radiation_on_Inclined_Surface3/2
  Radiation_on_Inclined_Surface3/1 -> Window_Optics3/1
  Fixed_Surface4/1 -> Radiation_on_Inclined_Surface4/2
  Radiation_on_Inclined_Surface4/1 -> Window_Optics4/1
  troom_calc/1(Troom) -> Troom/1, Sum4/1, Sum2/2  "Troom"
  window/1 -> Demux/1  "Qdot_trans_window"
  Demux1/4 -> Bus Creator/14  "Qdot_solar4"
  Demux1/1 -> Bus Creator/11  "Qdot_solar1"
  Demux1/2 -> Bus Creator/12  "Qdot_solar2"
  Demux1/3 -> Bus Creator/13  "Qdot_solar3"
  Demux/2 -> Bus Creator/4  "Qdot_trans_window2"
  Demux/3 -> Bus Creator/5  "Qdot_trans_window3"
  Demux/4 -> Bus Creator/6  "Qdot_trans_window4"

== system carnot/Basic/Thermal_Models/Pipe_basic ==
  Tamb : Inport
  THBin : Inport  Port=2
  Bus Assignment : BusAssignment  AssignedSignals=Temperature
  Bus Selector : BusSelector  OutputSignals=Temperature,MassFlow,Pressure,FluidType,FluidMix
  S-Function : S-Function  FunctionName=pipe_Tnodes  Parameters="vnode, lnode,  unode,  cond,  cnode,  t0, nodes"  EnableBusSupport=off
  Tnodes : Outport
  THB : Outport  Port=2
  wires:
  THBin/1 -> Bus Assignment/1, Bus Selector/1
  S-Function/1 -> Bus Assignment/2
  Tamb/1 -> S-Function/1
  Bus Selector/1 -> S-Function/2  "<Temperature>"
  Bus Selector/2 -> S-Function/3  "<MassFlow>"
  Bus Selector/3 -> S-Function/4  "<Pressure>"
  Bus Selector/4 -> S-Function/5  "<FluidType>"
  Bus Selector/5 -> S-Function/6  "<FluidMix>"
  S-Function/2 -> Tnodes/1
  Bus Assignment/1 -> THB/1

== system carnot/Basic/Thermal_Models/Radiator_basic ==
  note: One node model with upwind scheme. Power balance is:
      | m*cp*dTnode/dt = -qdot + mdot*cp*(Tin - Tnode)
      |
      | EN 442:
      | qdot = qdot_nominal * ((Tnode-Troom)/(Tdiff_nominal)^expo
      | nominal temperature difference = 50K with flowline 75°C, return 65°C and room 20°C
      | in EN, the Tnode is mean temperature Tm = 0.5*(Tin+Tout)
      |
      | Here Tout = Tnode in difference to EN442
      | A correction of expo and nominal power is done in the mask.
  THB_in : Inport
  Troom : Inport  Port=2
  1/(m*cp) : Gain  Gain=1/mcap  SaturateOnIntegerOverflow=on  OutDataTypeStr=Inherit: Same as input  ParamDataTypeStr=Inherit: Same as input
  Abs : Abs  SaturateOnIntegerOverflow=on
  Bus Selector : BusSelector  OutputSignals=Temperature,MassFlow
  Gain : Gain  Gain=1/dtnom  SaturateOnIntegerOverflow=on  OutDataTypeStr=Inherit: Same as input  ParamDataTypeStr=Inherit: Same as input
  Gain1 : Gain  Gain=pnom  SaturateOnIntegerOverflow=on  OutDataTypeStr=Inherit: Same as input  ParamDataTypeStr=Inherit: Same as input
  Heat_Capacity : carnot/Basic/Material_Properties/Heat_Capacity  VariantControl=CarlibClassic  INPUTARGUMENTS=THB  DEBUGLEVEL=DEBUGLEVEL  MAXTOTALWARNINGS=inf  MAXCONSECUTIVEWARNINGS=inf  WRITETOFILE=0  FILENAME='errors.txt'
  Math Function : Math  Operator=pow  SaturateOnIntegerOverflow=on
  Product : Product  Inputs=3  SaturateOnIntegerOverflow=on  InputSameDT=on  OutDataTypeStr=Inherit: Same as first input
  Product1 : Product  SaturateOnIntegerOverflow=on  InputSameDT=on  OutDataTypeStr=Inherit: Same as first input
  Sign : Signum
  Sum : Sum  Inputs=-+  SaturateOnIntegerOverflow=on  InputSameDT=on  OutDataTypeStr=Inherit: Same as first input
  Sum1 : Sum  Inputs=-+  SaturateOnIntegerOverflow=on  InputSameDT=on  OutDataTypeStr=Inherit: Same as first input
  Sum3 : Sum  Inputs=-+  SaturateOnIntegerOverflow=on  InputSameDT=on  OutDataTypeStr=Inherit: Same as first input
  THB_set_T : carnot/Source/Simple/THB_set_T
  Transfer Fcn (with initial states) : Subsystem  mask(Transfer Function with Initial States){N=[1], D=[1  0], X0=20}
      mask prompts: N "Numerator:"; D "Denominator:"; X0 "Initial conditions:"
      mask help: Vector expressions for numerator, and denominator. Coefficients are in descending powers of s.
      mask init:
      | [A,B,C,Dd]=tf2ss(N,D);if (isempty(X0));[m,n]=size(A);X0=zeros(1,m); end;
      mask Help: Specify the initial states for the transfer function.  The state ordering is determined by the m-file tf2ss.  There is no unique mapping of the states in a transfer function to states in a state-space representation.  However, tf2ss will consistently use the same mapping for a given transfer function.
      mask Display: dpoly(N,D,'s')
  const : Constant  Value=expo
  THB : Outport
  Qdot2room : Outport  Port=2
  wires:
  Troom/1 -> Sum3/1
  Bus Selector/1 -> Sum/2  "<Temperature>"
  Sign/1 -> Product1/2
  Sum3/1 -> Sign/1, Gain/1
  Gain1/1 -> Product1/1
  Abs/1 -> Math Function/1
  Gain/1 -> Abs/1
  Math Function/1 -> Gain1/1
  const/1 -> Math Function/2
  Product1/1 -> Qdot2room/1, Sum1/1
  Sum/1 -> Product/1
  Bus Selector/2 -> Product/2  "<MassFlow>"
  Heat_Capacity/1 -> Product/3
  Product/1 -> Sum1/2
  Sum1/1 -> 1/(m*cp)/1
  1/(m*cp)/1 -> Transfer Fcn (with initial states)/1(In1)
  Transfer Fcn (with initial states)/1(Out1) -> Sum3/2, Sum/1, THB_set_T/2
  THB_set_T/1 -> THB/1
  THB_in/1 -> Bus Selector/1, Heat_Capacity/1, THB_set_T/1

== system carnot/Basic/Thermal_Models/Solar_Collector_basic ==
  solar : Inport
  THB : Inport  Port=2
  Bus Selector1 : BusSelector  OutputSignals=Temperature,MassFlow
  Bus Selector2 : BusSelector  OutputSignals=Pressure,FluidType,FluidMix  OutputAsBus=on
  S-Function : S-Function  FunctionName=solarcollector12975  Parameters=acol, c1, c2, c3, c4, c5, c6, tini  EnableBusSupport=off
  Tout : Outport
  Tmean : Outport  Port=2
  Qdot : Outport  Port=3
  wires:
  Bus Selector1/2 -> S-Function/3  "<MassFlow>"
  Bus Selector1/1 -> S-Function/2  "<Temperature>"
  Bus Selector2/1 -> S-Function/4
  THB/1 -> Bus Selector1/1, Bus Selector2/1
  solar/1 -> S-Function/1
  S-Function/1 -> Tout/1  "Tout"
  S-Function/2 -> Tmean/1  "Tmean"
  S-Function/3 -> Qdot/1  "power"

== system carnot/Basic/Thermal_Models/T_Ground_Undisturbed ==
  note: u(1) - u(2)*exp(-u(3)/u(4))*cos(2*pi*(u(5)-u(6)*3600)/(365*24*3600) - u(3)/u(4)) + 0.03*u(3)
  -1/delta_grd : Gain  Gain=-1/delta_grd
  Math Function : Math  SaturateOnIntegerOverflow=on
  Product : Product  RndMeth=Zero
  Sine Wave : Sin  Amplitude=deltathetae  Frequency=2*pi/(365*24*3600)  Phase=pi/2 - 2*pi*tshift/(365*24) - z/delta_grd  SampleTime=0
  Sum : Sum  Inputs=+-+
  Tmeanoutside1 : Constant  Value=Tmeanoutside
  gain : Gain  Gain=0.03
  height vector : Constant  Value=z
  Tearth : Outport
  wires:
  Tmeanoutside1/1 -> Sum/1
  Sum/1 -> Tearth/1
  Product/1 -> Sum/2
  Sine Wave/1 -> Product/2
  Math Function/1 -> Product/1
  -1/delta_grd/1 -> Math Function/1
  height vector/1 -> -1/delta_grd/1, gain/1
  gain/1 -> Sum/3

== system carnot/Basic/Thermal_Models/Thermal_Capacity ==
  Tin : Inport
  mdot : Inport  Port=2
  1/(m*cp) : Gain  Gain=1/mcp  SaturateOnIntegerOverflow=on  OutDataTypeStr=Inherit: Same as input  ParamDataTypeStr=Inherit: Same as input
  Integrator : Integrator  InitialCondition=Tamb
  Losses : Gain  Gain=UA  SaturateOnIntegerOverflow=on  OutDataTypeStr=Inherit: Same as input  ParamDataTypeStr=Inherit: Same as input
  Product1 : Product  Inputs=3  SaturateOnIntegerOverflow=on  InputSameDT=on  OutDataTypeStr=Inherit: Same as first input
  Sum1 : Sum  Inputs=-+  SaturateOnIntegerOverflow=on  InputSameDT=on  OutDataTypeStr=Inherit: Same as first input
  Sum2 : Sum  Inputs=-+  SaturateOnIntegerOverflow=on  InputSameDT=on  OutDataTypeStr=Inherit: Same as first input
  Sum3 : Sum  Inputs=+-  SaturateOnIntegerOverflow=on  InputSameDT=on  OutDataTypeStr=Inherit: Same as first input
  Tamb : Constant  Value=Tamb
  cp_approx : Constant  Value=cp_approx
  Tout : Outport
  wires:
  mdot/1 -> Product1/2
  Tin/1 -> Sum1/2
  Integrator/1 -> Sum1/1, Sum3/1, Tout/1
  Product1/1 -> Sum2/2
  Sum2/1 -> 1/(m*cp)/1
  Tamb/1 -> Sum3/2
  Losses/1 -> Sum2/1
  Sum3/1 -> Losses/1
  cp_approx/1 -> Product1/3
  1/(m*cp)/1 -> Integrator/1
  Sum1/1 -> Product1/1

== system carnot/Basic/Thermal_Models/Thermal_Node ==
  Tamb : Inport
  Tin : Inport  Port=2
  mdot : Inport  Port=3
  Qdot : Inport  Port=4
  1/(m*cp) : Gain  Gain=1/mcp  SaturateOnIntegerOverflow=on  OutDataTypeStr=Inherit: Same as input  ParamDataTypeStr=Inherit: Same as input
  Integrator : Integrator  InitialCondition=Tini
  Losses : Gain  Gain=UA  SaturateOnIntegerOverflow=on  OutDataTypeStr=Inherit: Same as input  ParamDataTypeStr=Inherit: Same as input
  Product1 : Product  Inputs=3  SaturateOnIntegerOverflow=on  InputSameDT=on  OutDataTypeStr=Inherit: Same as first input
  Sum1 : Sum  Inputs=-+  SaturateOnIntegerOverflow=on  InputSameDT=on  OutDataTypeStr=Inherit: Same as first input
  Sum2 : Sum  Inputs=-++  SaturateOnIntegerOverflow=on  InputSameDT=on  OutDataTypeStr=Inherit: Same as first input
  Sum3 : Sum  Inputs=+-  SaturateOnIntegerOverflow=on  InputSameDT=on  OutDataTypeStr=Inherit: Same as first input
  Sum4 : Sum  Inputs=1  SaturateOnIntegerOverflow=on  InputSameDT=on  OutDataTypeStr=Inherit: Same as first input
  cp_approx : Constant  Value=cp_approx
  Tout : Outport
  wires:
  Qdot/1 -> Sum4/1
  mdot/1 -> Product1/2
  Tin/1 -> Sum1/2
  Integrator/1 -> Sum1/1, Sum3/1, Tout/1
  Product1/1 -> Sum2/2
  Sum2/1 -> 1/(m*cp)/1
  Tamb/1 -> Sum3/2
  Losses/1 -> Sum2/1
  Sum3/1 -> Losses/1
  cp_approx/1 -> Product1/3
  1/(m*cp)/1 -> Integrator/1
  Sum1/1 -> Product1/1
  Sum4/1 -> Sum2/3

== system carnot/Basic/Thermal_Models/Wall_basic ==
  qdot_in : Inport
  QdotActive : Inport  Port=2
  qdot_out : Inport  Port=3
  S-Function : S-Function  FunctionName=layerwall  Parameters=tau, t0, d, cond, cwall, rho, dactive  EnableBusSupport=off
  Tin : Outport
  Tactive : Outport  Port=2
  Tout : Outport  Port=3
  wires:
  qdot_in/1 -> S-Function/1
  S-Function/1 -> Tin/1
  QdotActive/1 -> S-Function/2
  S-Function/2 -> Tactive/1  "T(active)"
  qdot_out/1 -> S-Function/3
  S-Function/3 -> Tout/1

== system carnot/Basic/Thermal_Models/sfun_storageTnodes ==
  Tamb : Inport
  port1 : Inport  Port=2
  port2 : Inport  Port=3
  port3 : Inport  Port=4
  port4 : Inport  Port=5
  port5 : Inport  Port=6
  port6 : Inport  Port=7
  port7 : Inport  Port=8
  port8 : Inport  Port=9
  port9 : Inport  Port=10
  port10 : Inport  Port=11
  sfun_storageTnodes : S-Function  FunctionName=storage_Tnodes  Parameters=dia, volume, standing, uloss , ubot, utop, cond, tini, nodes, nconnect  EnableBusSupport=off
  Energy : Outport
  Tnodes : Outport  Port=2
  wires:
  port10/1 -> sfun_storageTnodes/11
  port9/1 -> sfun_storageTnodes/10
  port8/1 -> sfun_storageTnodes/9
  port7/1 -> sfun_storageTnodes/8
  port6/1 -> sfun_storageTnodes/7
  port5/1 -> sfun_storageTnodes/6
  port4/1 -> sfun_storageTnodes/5
  port3/1 -> sfun_storageTnodes/4
  port2/1 -> sfun_storageTnodes/3
  port1/1 -> sfun_storageTnodes/2
  Tamb/1 -> sfun_storageTnodes/1
  sfun_storageTnodes/2 -> Tnodes/1
  sfun_storageTnodes/1 -> Energy/1
